simulink model "lab5"  (R2021b)
settings: Solver=FixedStepAuto  StartTime=0.0  StopTime=120  FixedStep=0.01  RelTol=1e-3
model workspace (MAT data in the model file):
  Ti = 200
values from neighbouring files (symbols this model uses):
  ddMax = 3    [sysdata.m]
  deltaMax = 30    [sysdata.m]
  fConst = 0    [sysdata.m]
  K = 0.08    [sysdata.m]
  Kc = 0.7045    [sysdata.m]
  phiZad = 30    [sysdata.m]
  Toc = 5    [sysdata.m]
  Tr = 1    [sysdata.m]
  Ts = 18    [sysdata.m]
settings Model: Creator=valeria  LastModifiedBy=Ivan
settings SolverCC: AlgebraicLoopSolver=TrustRegion
settings DebuggingCC: SFMachineParentedDataDiag=warning

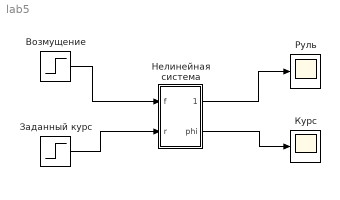
== system lab5 ==
  Возмущение : Step  Time=0  After=fConst  SampleTime=0
  Заданный курс : Step  Time=0  After=phiZad  SampleTime=0
  Курс : Scope
  Нелинейная система : Subsystem
  Руль : Scope
  wires:
  Возмущение/1 -> Нелинейная система/1(f)
  Заданный курс/1 -> Нелинейная система/2(r)
  Нелинейная система/1(delta) -> Руль/1
  Нелинейная система/2(phi) -> Курс/1

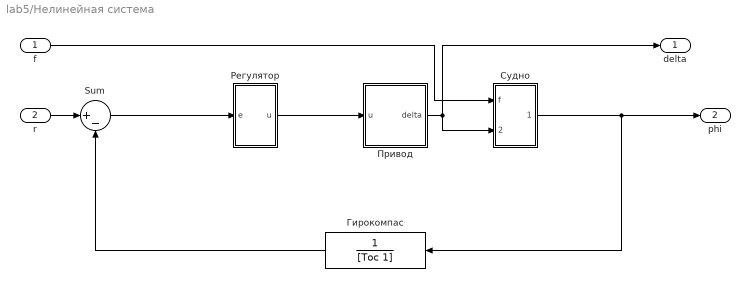
== system lab5/Нелинейная система ==
  f : Inport
  r : Inport  Port=2
  " Гирокомпас" : TransferFcn  Denominator=[Toc 1]
  Sum : Sum  Inputs=|+-
  Привод : Subsystem
  Регулятор : Subsystem
  Судно : Subsystem
  delta : Outport
  phi : Outport  Port=2
  wires:
  r/1 -> Sum/1
  Судно/1(phi) -> phi/1, " Гирокомпас"/1
  " Гирокомпас"/1 -> Sum/2
  Привод/1(delta) -> delta/1, Судно/2(delta)
  f/1 -> Судно/1(f)
  Sum/1 -> Регулятор/1(e)
  Регулятор/1(u) -> Привод/1(u)

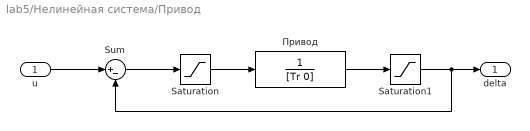
== system lab5/Нелинейная система/Привод ==
  u : Inport
  Saturation : Saturate  UpperLimit=+ddMax  LowerLimit=-ddMax
  Saturation1 : Saturate  UpperLimit=+deltaMax  LowerLimit=-deltaMax
  Sum : Sum  Inputs=|+-
  Привод : TransferFcn  Denominator=[Tr 0]
  delta : Outport
  wires:
  u/1 -> Sum/1
  Sum/1 -> Saturation/1
  Saturation/1 -> Привод/1
  Привод/1 -> Saturation1/1
  Saturation1/1 -> Sum/2, delta/1

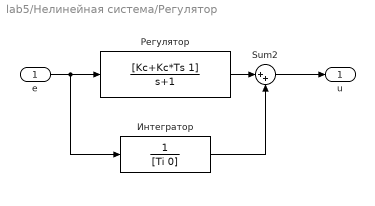
== system lab5/Нелинейная система/Регулятор ==
  e : Inport
  " Интегратор" : TransferFcn  Denominator=[Ti 0]
  Sum2 : Sum  Inputs=|++
  Регулятор : TransferFcn  Numerator=[Kc+Kc*Ts 1]  Denominator=[1 1]
  u : Outport
  wires:
  " Интегратор"/1 -> Sum2/2
  e/1 -> " Интегратор"/1, Регулятор/1
  Регулятор/1 -> Sum2/1
  Sum2/1 -> u/1

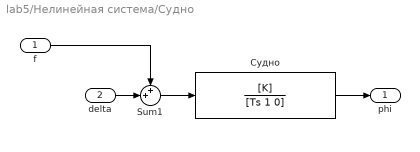
== system lab5/Нелинейная система/Судно ==
  f : Inport
  delta : Inport  Port=2
  Sum1 : Sum  Inputs=++|
  Судно : TransferFcn  Numerator=[K]  Denominator=[Ts 1 0]
  phi : Outport
  wires:
  Sum1/1 -> Судно/1
  Судно/1 -> phi/1
  delta/1 -> Sum1/2
  f/1 -> Sum1/1
